simulink model "main_train_proto_zd_rt_actualizado_discrete"  (Simulink 7.8)
settings: Solver=ode45  StartTime=0.0  StopTime=50  RelTol=1e-3
settings Model: Creator=imac  LastModifiedBy=aitor
settings DebuggingCC: FcnCallInpInsideContextMsg=Use local settings

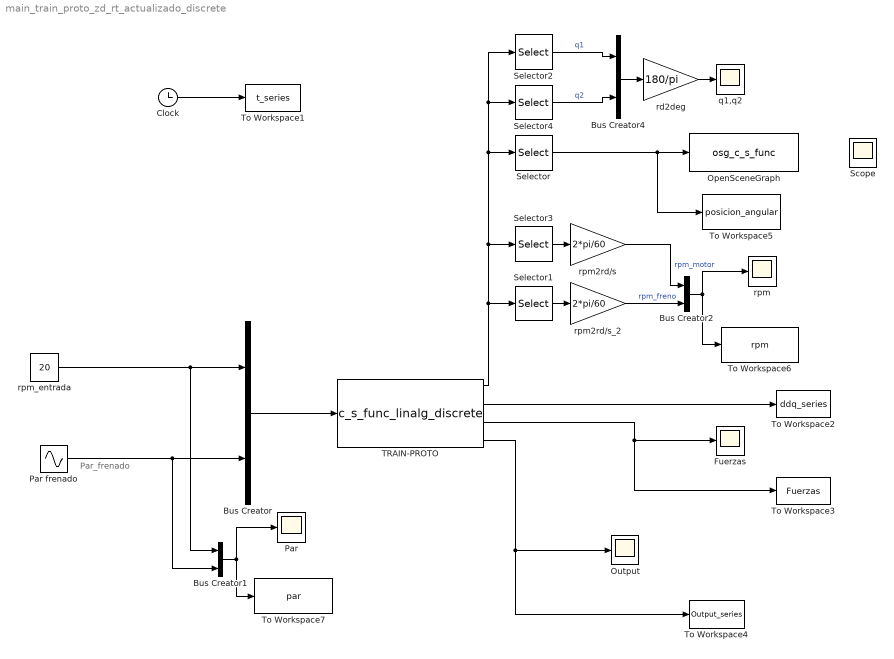
== system main_train_proto_zd_rt_actualizado_discrete ==
  note: Par_frenado
  Bus Creator{,1..2,4} (4 alike) : BusCreator  Inputs=2
  Clock : Clock
  Fuerzas : Scope
      settings: TimeRange=50  YMin=274.2  YMax=275.7  SaveName=ScopeData2  SampleInput=on  SampleTime=0.01
  OpenSceneGraph : S-Function  FunctionName=osg_c_s_func  EnableBusSupport=off
  Output : Scope
      settings: YMin=-70  YMax=20  SaveName=ScopeData3  SampleInput=on  SampleTime=0.01
  Par : Scope
      settings: TimeRange=50  YMin=5  YMax=25
  Par frenado : Sin  Amplitude=10  Bias=15  Phase=pi/2  SampleTime=0
  Scope : Scope
      settings: SaveName=ScopeData4
  Selector : Selector  InputPortWidth=12  IndexOptions=Index vector (dialog)  Indices=[1 2 3 4 5 6]  OutputSizes=1
  Selector1 : Selector  InputPortWidth=12  IndexOptions=Index vector (dialog)  Indices=[9]  OutputSizes=1
  Selector2 : Selector  InputPortWidth=12  IndexOptions=Index vector (dialog)  Indices=[1]  OutputSizes=1
  Selector3 : Selector  InputPortWidth=12  IndexOptions=Index vector (dialog)  Indices=[11]  OutputSizes=1
  Selector4 : Selector  InputPortWidth=12  IndexOptions=Index vector (dialog)  Indices=[2]  OutputSizes=1
  TRAIN-PROTO : S-Function  FunctionName=c_s_func_linalg_discrete  Parameters=q dq param Delta_t  EnableBusSupport=off
      mask Type: S-function: mycsfunc
      mask Description: This is a S-function that does the continuous state space system.
      mask Display: disp('[M , Phi_q''] [ddq]\n[Phi_q , 0] [lambda]\n=\n [Q ] \n   [gamma] ');
  To Workspace1 : ToWorkspace  VariableName=t_series  SampleTime=0.01  SaveFormat=Array
  To Workspace2 : ToWorkspace  VariableName=ddq_series  SampleTime=0.01  SaveFormat=Array
  To Workspace3 : ToWorkspace  VariableName=Fuerzas  SampleTime=-1  SaveFormat=Structure With Time
  To Workspace4 : ToWorkspace  VariableName=Output_series  SampleTime=0.01  SaveFormat=Array
  To Workspace5 : ToWorkspace  VariableName=posicion_angular  SampleTime=-1  SaveFormat=Structure With Time
  To Workspace6 : ToWorkspace  VariableName=rpm  SampleTime=-1  SaveFormat=Structure With Time
  To Workspace7 : ToWorkspace  VariableName=par  SampleTime=-1  SaveFormat=Structure With Time
  q1,q2 : Scope
      settings: TimeRange=50  YMin=-3  YMax=3  SampleInput=on  SampleTime=0.01
  rd2deg : Gain  Gain=180/pi
  rpm : Scope
      settings: TimeRange=50  YMin=-200  YMax=200  SaveName=ScopeData5  SampleInput=on  SampleTime=0.01
  rpm2rd/s : Gain  Gain=2*pi/60
  rpm2rd/s_2 : Gain  Gain=2*pi/60
  rpm_entrada : Constant  Value=20
  wires:
  Clock/1 -> To Workspace1/1
  TRAIN-PROTO/1 -> Selector3/1, Selector/1, Selector2/1, Selector4/1, Selector1/1
  TRAIN-PROTO/2 -> To Workspace2/1
  TRAIN-PROTO/3 -> To Workspace3/1, Fuerzas/1
  TRAIN-PROTO/4 -> Output/1, To Workspace4/1
  Selector/1 -> OpenSceneGraph/1, To Workspace5/1
  ? -> Scope/1
  Bus Creator/1 -> TRAIN-PROTO/1
  Par frenado/1 -> Bus Creator/2, Bus Creator1/2
  rpm_entrada/1 -> Bus Creator/1, Bus Creator1/1
  Selector2/1 -> Bus Creator4/1  "q1"
  Selector4/1 -> Bus Creator4/2  "q2"
  Bus Creator4/1 -> rd2deg/1
  rd2deg/1 -> q1,q2/1
  rpm2rd/s/1 -> Bus Creator2/1  "rpm_motor"
  Selector1/1 -> rpm2rd/s_2/1
  rpm2rd/s_2/1 -> Bus Creator2/2  "rpm_freno"
  Bus Creator2/1 -> To Workspace6/1, rpm/1
  Selector3/1 -> rpm2rd/s/1
  Bus Creator1/1 -> To Workspace7/1, Par/1
